simulink model "kumaraGazeboSim2019"  (R2019b)
settings: Solver=FixedStepAuto  StartTime=0.0  StopTime=inf  RelTol=1e-3
model workspace (MAT data in the model file):
  SL_ROS_VariableLengthArrays_MaxSizes.CommonInfo.ArrayTruncateAction = 'EmitWarning'
  SL_ROS_VariableLengthArrays_MaxSizes.MsgTypeMap = containers.Map
  SL_ROS_VariableLengthArrays_MaxSizes.MsgTypeMap.serialization.keys = {'gazebo_msgs/LinkState', 'sensor_msgs/JointState'}
  SL_ROS_VariableLengthArrays_MaxSizes.MsgTypeMap.serialization.values{1}(1).PropertyName = 'LinkName'
  SL_ROS_VariableLengthArrays_MaxSizes.MsgTypeMap.serialization.values{1}(1).DataType = 'uint8'
  SL_ROS_VariableLengthArrays_MaxSizes.MsgTypeMap.serialization.values{1}(1).MaxLength = 18
  SL_ROS_VariableLengthArrays_MaxSizes.MsgTypeMap.serialization.values{1}(2).PropertyName = 'ReferenceFrame'
  SL_ROS_VariableLengthArrays_MaxSizes.MsgTypeMap.serialization.values{1}(2).DataType = 'uint8'
  SL_ROS_VariableLengthArrays_MaxSizes.MsgTypeMap.serialization.values{1}(2).MaxLength = 22
  SL_ROS_VariableLengthArrays_MaxSizes.MsgTypeMap.serialization.values{2}(1).PropertyName = 'Effort'
  SL_ROS_VariableLengthArrays_MaxSizes.MsgTypeMap.serialization.values{2}(1).DataType = 'double'
  SL_ROS_VariableLengthArrays_MaxSizes.MsgTypeMap.serialization.values{2}(1).MaxLength = 13
  SL_ROS_VariableLengthArrays_MaxSizes.MsgTypeMap.serialization.values{2}(2).PropertyName = 'Name'
  SL_ROS_VariableLengthArrays_MaxSizes.MsgTypeMap.serialization.values{2}(2).DataType = 'std_msgs/String'
  SL_ROS_VariableLengthArrays_MaxSizes.MsgTypeMap.serialization.values{2}(2).MaxLength = 13
  SL_ROS_VariableLengthArrays_MaxSizes.MsgTypeMap.serialization.values{2}(3).PropertyName = 'Position'
  SL_ROS_VariableLengthArrays_MaxSizes.MsgTypeMap.serialization.values{2}(3).DataType = 'double'
  SL_ROS_VariableLengthArrays_MaxSizes.MsgTypeMap.serialization.values{2}(3).MaxLength = 13
  SL_ROS_VariableLengthArrays_MaxSizes.MsgTypeMap.serialization.values{2}(4).PropertyName = 'Velocity'
  SL_ROS_VariableLengthArrays_MaxSizes.MsgTypeMap.serialization.values{2}(4).DataType = 'double'
  SL_ROS_VariableLengthArrays_MaxSizes.MsgTypeMap.serialization.values{2}(4).MaxLength = 13
  SL_ROS_VariableLengthArrays_MaxSizes.MsgTypeMap.serialization.uniformity = 0
  SL_ROS_VariableLengthArrays_MaxSizes.MsgTypeMap.serialization.keyType = 'char'
  SL_ROS_VariableLengthArrays_MaxSizes.MsgTypeMap.serialization.valueType = 'any'
libraries: robotlib x21, simulink x3, simulink_extras x2
settings Model: EnablePacing=on  Creator=pokpong.c  LastModifiedBy=pokpong.c
settings OptimizationCC: EnhancedBackFolding=on  PassReuseOutputArgsAs=Individual arguments  ZeroExternalMemoryAtStartup=off  ZeroInternalMemoryAtStartup=off  MaxStackSize=64  OptimizeBlockOrder=speed  DifferentSizesBufferReuse=on  OptimizationCustomize=off  EfficientTunableParamExpr=on
settings DebuggingCC: ParameterTunabilityLossMsg=error
settings HardwareCC: ProdBitPerPointer=32  ProdBitPerSizeT=32  ProdBitPerPtrDiffT=32  ProdLargestAtomicFloat=None  ProdIntDivRoundTo=Undefined  ProdEndianess=Unspecified  ProdWordSize=32  ProdHWDeviceType=Generic->Unspecified (assume 32-bit Generic)
settings SFSimCC: MATLABDynamicMemAlloc=off
settings RTWCC: SystemTargetFile=ert.tlc  HardwareBoard=Robot Operating System (ROS)  TLCOptions="-aInlineSetEventsForThisBaseRateFcn=TLC_FALSE -aSuppressMultiTaskScheduler=TLC_FALSE  -aRateBasedStepFcn=0"  TemplateMakefile=ert_default_tmf  Toolchain=Catkin  TargetLang=C++
settings CodeAppCC: ForceParamTrailComments=on  IgnoreCustomStorageClasses=off  OperatorAnnotations=on  SimulinkDataObjDesc=on  SFDataObjDesc=on  InsertBlockDesc=on

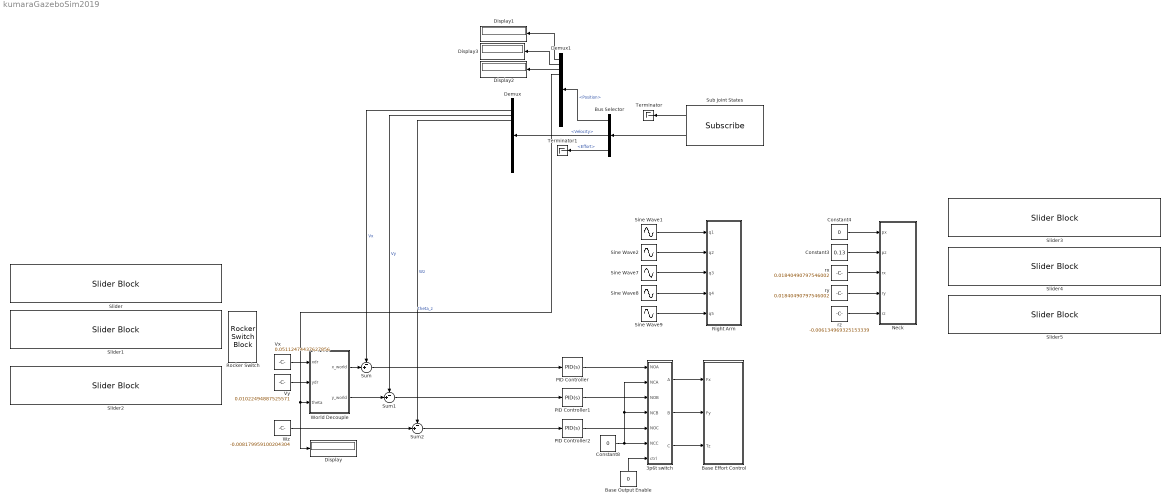
== system kumaraGazeboSim2019 ==
  3p6t switch : Subsystem
  Base Effort Control : Subsystem
  Base Output Enable : Constant  Value=0
  Bus Selector : BusSelector  OutputSignals=Position,Velocity,Effort
  Constant3 : Constant  Value=0.13
  Constant4 : Constant  Value=0
  Constant8 : Constant  Value=0
  Demux : Demux  Outputs=13
  Demux1 : Demux  Outputs=13
  Display{,1..3} (4 alike) : Display
  Neck : Subsystem
  PID Controller : simulink/Continuous/PID Controller  Controller=PID  Form=Parallel  TimeDomain=Continuous-time  SampleTime=-1  IntegratorMethod=Forward Euler  FilterMethod=Forward Euler  ControllerParametersSource=internal  P=40  I=1  D=0  UseFilter=on  N=100  TunerSelectOption=Transfer Function Based (PID Tuner App)  InitialConditionSource=internal  InitialConditionForIntegrator=0  InitialConditionForFilter=0  DifferentiatorICPrevScaledInput=0  ExternalReset=none  TrackingMode=off  Kt=1  LimitOutput=off  UpperSaturationLimit=inf  LowerSaturationLimit=-inf  LinearizeAsGain=on  AntiWindupMode=none  Kb=1  POutMin=[]  POutMax=[]  IOutMin=[]  IOutMax=[]  DOutMin=[]  DOutMax=[]  NOutMin=[]  NOutMax=[]  SumOutMin=[]  SumOutMax=[]  SaturationOutMin=[]  SaturationOutMax=[]  PParamMin=[]  PParamMax=[]  IParamMin=[]  IParamMax=[]  DParamMin=[]  DParamMax=[]  NParamMin=[]  NParamMax=[]  KbParamMin=[]  KbParamMax=[]  KtParamMin=[]  KtParamMax=[]  KbOutMin=[]  KbOutMax=[]  KtOutMin=[]  KtOutMax=[]  IntegratorOutMin=[]  IntegratorOutMax=[]  FilterOutMin=[]  FilterOutMax=[]  SumI1OutMin=[]  SumI1OutMax=[]  SumI2OutMin=[]  SumI2OutMax=[]  SumI3OutMin=[]  SumI3OutMax=[]  SumI4OutMin=[]  SumI4OutMax=[]  SumDOutMin=[]  SumDOutMax=[]  DifferentiatorOutMin=[]  DifferentiatorOutMax=[]  FilterDiffOutCoefMin=[]  FilterDiffOutCoefMax=[]  ReciprocalOutMin=[]  ReciprocalOutMax=[]  SumDenOutMin=[]  SumDenOutMax=[]  SumNumOutMin=[]  SumNumOutMax=[]  DivideOutMin=[]  DivideOutMax=[]  IntegratorContinuousStateAttributes=''  IntegratorStateMustResolveToSignalObject=off  IntegratorRTWStateStorageClass=Auto  FilterContinuousStateAttributes=''  FilterStateMustResolveToSignalObject=off  FilterRTWStateStorageClass=Auto  ParallelPVariant=InternalParameters  IdealPVariant=Disabled  IVariant=InternalParameters  DVariant=InternalParameters  IntegratorVariant=Continuous  SatVariant=Disabled  AWVariant=Passthrough  PCopyVariant=Disabled  TRVariant=Disabled  FdbkBlocksVariant=Forward  IdealPFdbkVariant=Disabled  SatFdbkVariant=Disabled  DerivativeFilterVariant=ContFilter  NVariant=InternalParameters  NCopyVariant=Disabled  FilterICVariant=InternalICsFilter  IntegratorICVariant=InternalICs  ExternalResetVariant=Disabled  TRSumVariant=Passthrough  SumFdbkVariant=Disabled  SumVariant=Sum_PID
  PID Controller1 : simulink/Continuous/PID Controller  Controller=PID  Form=Parallel  TimeDomain=Continuous-time  SampleTime=-1  IntegratorMethod=Forward Euler  FilterMethod=Forward Euler  ControllerParametersSource=internal  P=40  I=1  D=0  UseFilter=on  N=100  TunerSelectOption=Transfer Function Based (PID Tuner App)  InitialConditionSource=internal  InitialConditionForIntegrator=0  InitialConditionForFilter=0  DifferentiatorICPrevScaledInput=0  ExternalReset=none  TrackingMode=off  Kt=1  LimitOutput=off  UpperSaturationLimit=inf  LowerSaturationLimit=-inf  LinearizeAsGain=on  AntiWindupMode=none  Kb=1  POutMin=[]  POutMax=[]  IOutMin=[]  IOutMax=[]  DOutMin=[]  DOutMax=[]  NOutMin=[]  NOutMax=[]  SumOutMin=[]  SumOutMax=[]  SaturationOutMin=[]  SaturationOutMax=[]  PParamMin=[]  PParamMax=[]  IParamMin=[]  IParamMax=[]  DParamMin=[]  DParamMax=[]  NParamMin=[]  NParamMax=[]  KbParamMin=[]  KbParamMax=[]  KtParamMin=[]  KtParamMax=[]  KbOutMin=[]  KbOutMax=[]  KtOutMin=[]  KtOutMax=[]  IntegratorOutMin=[]  IntegratorOutMax=[]  FilterOutMin=[]  FilterOutMax=[]  SumI1OutMin=[]  SumI1OutMax=[]  SumI2OutMin=[]  SumI2OutMax=[]  SumI3OutMin=[]  SumI3OutMax=[]  SumI4OutMin=[]  SumI4OutMax=[]  SumDOutMin=[]  SumDOutMax=[]  DifferentiatorOutMin=[]  DifferentiatorOutMax=[]  FilterDiffOutCoefMin=[]  FilterDiffOutCoefMax=[]  ReciprocalOutMin=[]  ReciprocalOutMax=[]  SumDenOutMin=[]  SumDenOutMax=[]  SumNumOutMin=[]  SumNumOutMax=[]  DivideOutMin=[]  DivideOutMax=[]  IntegratorContinuousStateAttributes=''  IntegratorStateMustResolveToSignalObject=off  IntegratorRTWStateStorageClass=Auto  FilterContinuousStateAttributes=''  FilterStateMustResolveToSignalObject=off  FilterRTWStateStorageClass=Auto  ParallelPVariant=InternalParameters  IdealPVariant=Disabled  IVariant=InternalParameters  DVariant=InternalParameters  IntegratorVariant=Continuous  SatVariant=Disabled  AWVariant=Passthrough  PCopyVariant=Disabled  TRVariant=Disabled  FdbkBlocksVariant=Forward  IdealPFdbkVariant=Disabled  SatFdbkVariant=Disabled  DerivativeFilterVariant=ContFilter  NVariant=InternalParameters  NCopyVariant=Disabled  FilterICVariant=InternalICsFilter  IntegratorICVariant=InternalICs  ExternalResetVariant=Disabled  TRSumVariant=Passthrough  SumFdbkVariant=Disabled  SumVariant=Sum_PID
  PID Controller2 : simulink/Continuous/PID Controller  Controller=PID  Form=Parallel  TimeDomain=Continuous-time  SampleTime=-1  IntegratorMethod=Forward Euler  FilterMethod=Forward Euler  ControllerParametersSource=internal  P=40  I=1  D=0  UseFilter=on  N=100  TunerSelectOption=Transfer Function Based (PID Tuner App)  InitialConditionSource=internal  InitialConditionForIntegrator=0  InitialConditionForFilter=0  DifferentiatorICPrevScaledInput=0  ExternalReset=none  TrackingMode=off  Kt=1  LimitOutput=off  UpperSaturationLimit=inf  LowerSaturationLimit=-inf  LinearizeAsGain=on  AntiWindupMode=none  Kb=1  POutMin=[]  POutMax=[]  IOutMin=[]  IOutMax=[]  DOutMin=[]  DOutMax=[]  NOutMin=[]  NOutMax=[]  SumOutMin=[]  SumOutMax=[]  SaturationOutMin=[]  SaturationOutMax=[]  PParamMin=[]  PParamMax=[]  IParamMin=[]  IParamMax=[]  DParamMin=[]  DParamMax=[]  NParamMin=[]  NParamMax=[]  KbParamMin=[]  KbParamMax=[]  KtParamMin=[]  KtParamMax=[]  KbOutMin=[]  KbOutMax=[]  KtOutMin=[]  KtOutMax=[]  IntegratorOutMin=[]  IntegratorOutMax=[]  FilterOutMin=[]  FilterOutMax=[]  SumI1OutMin=[]  SumI1OutMax=[]  SumI2OutMin=[]  SumI2OutMax=[]  SumI3OutMin=[]  SumI3OutMax=[]  SumI4OutMin=[]  SumI4OutMax=[]  SumDOutMin=[]  SumDOutMax=[]  DifferentiatorOutMin=[]  DifferentiatorOutMax=[]  FilterDiffOutCoefMin=[]  FilterDiffOutCoefMax=[]  ReciprocalOutMin=[]  ReciprocalOutMax=[]  SumDenOutMin=[]  SumDenOutMax=[]  SumNumOutMin=[]  SumNumOutMax=[]  DivideOutMin=[]  DivideOutMax=[]  IntegratorContinuousStateAttributes=''  IntegratorStateMustResolveToSignalObject=off  IntegratorRTWStateStorageClass=Auto  FilterContinuousStateAttributes=''  FilterStateMustResolveToSignalObject=off  FilterRTWStateStorageClass=Auto  ParallelPVariant=InternalParameters  IdealPVariant=Disabled  IVariant=InternalParameters  DVariant=InternalParameters  IntegratorVariant=Continuous  SatVariant=Disabled  AWVariant=Passthrough  PCopyVariant=Disabled  TRVariant=Disabled  FdbkBlocksVariant=Forward  IdealPFdbkVariant=Disabled  SatFdbkVariant=Disabled  DerivativeFilterVariant=ContFilter  NVariant=InternalParameters  NCopyVariant=Disabled  FilterICVariant=InternalICsFilter  IntegratorICVariant=InternalICs  ExternalResetVariant=Disabled  TRSumVariant=Passthrough  SumFdbkVariant=Disabled  SumVariant=Sum_PID
  Right Arm : Subsystem
  Rocker Switch : RockerSwitchBlock
      settings: Values={{'Off', 'On'}, [0 1]}
  Sine Wave{1..2,7..9} (5 alike) : Sin  Amplitude=3  Frequency=3  SampleTime=0
  Slider : SliderBlock  ScaleMin=-5  ScaleMax=5
  Slider1 : SliderBlock  ScaleMin=-5  ScaleMax=5
  Slider2 : SliderBlock  ScaleMin=-4  ScaleMax=4
  Slider3 : SliderBlock  ScaleMin=-3  ScaleMax=3
  Slider4 : SliderBlock  ScaleMin=-3  ScaleMax=3
  Slider5 : SliderBlock  ScaleMin=-3  ScaleMax=3
  Sub Joint States : robotlib/Subscribe  topicSource=Select from ROS network  topic=/kumara/joint_states  messageType=sensor_msgs/JointState  sampleTime=0.01  messageQueueLength=1
  Sum : Sum  Inputs=-+|
  Sum1 : Sum  Inputs=-+|
  Sum2 : Sum  Inputs=-+|
  Terminator : Terminator
  Terminator1 : Terminator
  Vx : Constant  Value=0.05112474437627856
  Vy : Constant  Value=0.01022494887525571
  World Decouple : Subsystem
  Wz : Constant  Value=-0.008179959100204304
  rx : Constant  Value=0.01840490797546002
  ry : Constant  Value=0.01840490797546002
  rz : Constant  Value=-0.006134969325153339
  wires:
  Vx/1 -> World Decouple/1("xdr ")
  Bus Selector/1 -> Demux1/1  "<Position>"
  Demux1/4 -> Display/1, World Decouple/3("theta ")  "theta_z"
  World Decouple/1(x_world) -> Sum/2
  World Decouple/2(y_world) -> Sum1/2
  PID Controller/1 -> 3p6t switch/1(NOA)
  Demux/4 -> Sum2/1  "Wz"
  Sum/1 -> PID Controller/1
  Base Output Enable/1 -> 3p6t switch/7(ctrl)
  Constant8/1 -> 3p6t switch/6(NCC), 3p6t switch/4(NCB), 3p6t switch/2(NCA)
  3p6t switch/1(A) -> Base Effort Control/1(Fx)
  Sub Joint States/2 -> Bus Selector/1
  Bus Selector/2 -> Demux/1  "<Velocity>"
  Vy/1 -> World Decouple/2(ydr)
  3p6t switch/3(C) -> Base Effort Control/3(Tz)
  Sum2/1 -> PID Controller2/1
  PID Controller1/1 -> 3p6t switch/3(NOB)
  Demux/3 -> Sum1/1  "Vy"
  Demux/2 -> Sum/1  "Vx"
  PID Controller2/1 -> 3p6t switch/5(NOC)
  Wz/1 -> Sum2/2
  Sum1/1 -> PID Controller1/1
  Sub Joint States/1 -> Terminator/1
  3p6t switch/2(B) -> Base Effort Control/2(Fy)
  Bus Selector/3 -> Terminator1/1  "<Effort>"
  Constant3/1 -> Neck/2(pz)
  Demux1/1 -> Display1/1
  Demux1/3 -> Display2/1
  Demux1/2 -> Display3/1
  Sine Wave1/1 -> Right Arm/1(q1)
  Sine Wave2/1 -> Right Arm/2(q2)
  Sine Wave7/1 -> Right Arm/3(q3)
  Sine Wave8/1 -> Right Arm/4(q4)
  Sine Wave9/1 -> Right Arm/5(q5)
  Constant4/1 -> Neck/1(px)
  rx/1 -> Neck/3(rx)
  ry/1 -> Neck/4(ry)
  rz/1 -> Neck/5(rz)

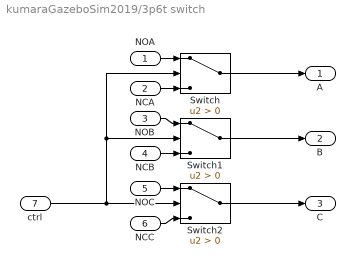
== system kumaraGazeboSim2019/3p6t switch ==
  NOA : Inport
  NCA : Inport  Port=2
  NOB : Inport  Port=3
  NCB : Inport  Port=4
  NOC : Inport  Port=5
  NCC : Inport  Port=6
  ctrl : Inport  Port=7
  Switch : Switch  Criteria=u2 > Threshold
  Switch1 : Switch  Criteria=u2 > Threshold
  Switch2 : Switch  Criteria=u2 > Threshold
  A : Outport
  B : Outport  Port=2
  C : Outport  Port=3
  wires:
  Switch1/1 -> B/1
  NCB/1 -> Switch1/3
  Switch/1 -> A/1
  NCC/1 -> Switch2/3
  Switch2/1 -> C/1
  ctrl/1 -> Switch2/2, Switch/2, Switch1/2
  NOA/1 -> Switch/1
  NOB/1 -> Switch1/1
  NCA/1 -> Switch/3
  NOC/1 -> Switch2/1

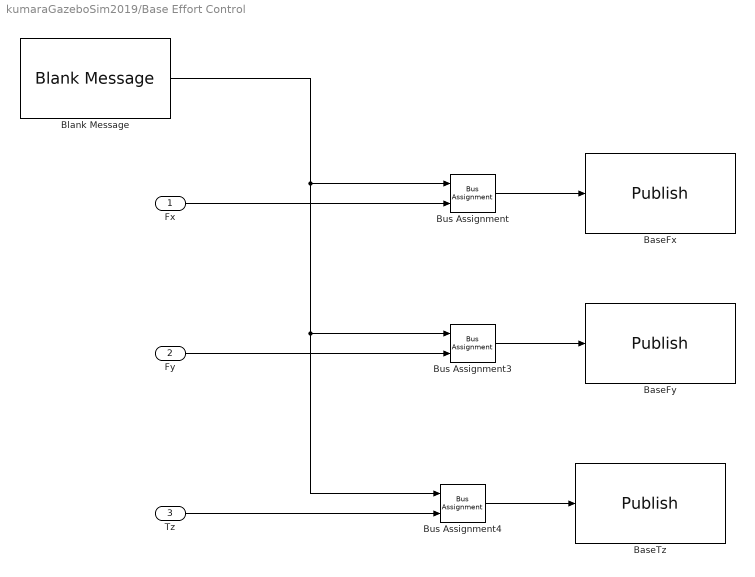
== system kumaraGazeboSim2019/Base Effort Control ==
  Fx : Inport
  Fy : Inport  Port=2
  Tz : Inport  Port=3
  BaseFx : robotlib/Publish  topicSource=Select from ROS network  topic=/kumara/base_x_force_controller/command  messageType=std_msgs/Float64  messageQueueLength=1
  BaseFy : robotlib/Publish  topicSource=Select from ROS network  topic=/kumara/base_y_force_controller/command  messageType=std_msgs/Float64  messageQueueLength=1
  BaseTz : robotlib/Publish  topicSource=Select from ROS network  topic=/kumara/base_z_torque_controller/command  messageType=std_msgs/Float64  messageQueueLength=1
  Blank Message : robotlib/Blank Message  messageClass=Message  entityType=std_msgs/Float64  messageType=std_msgs/Float64  SampleTime=inf
  Bus Assignment : BusAssignment  AssignedSignals=Data
  Bus Assignment3 : BusAssignment  AssignedSignals=Data
  Bus Assignment4 : BusAssignment  AssignedSignals=Data
  wires:
  Bus Assignment/1 -> BaseFx/1
  Bus Assignment3/1 -> BaseFy/1
  Bus Assignment4/1 -> BaseTz/1
  Blank Message/1 -> Bus Assignment/1, Bus Assignment3/1, Bus Assignment4/1
  Tz/1 -> Bus Assignment4/2
  Fx/1 -> Bus Assignment/2
  Fy/1 -> Bus Assignment3/2

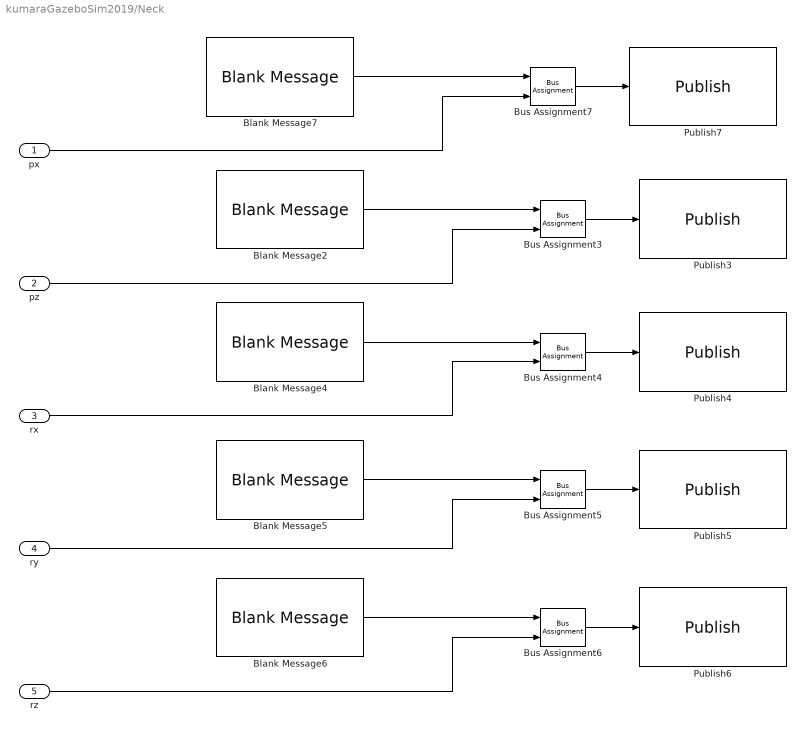
== system kumaraGazeboSim2019/Neck ==
  px : Inport
  pz : Inport  Port=2
  rx : Inport  Port=3
  ry : Inport  Port=4
  rz : Inport  Port=5
  Blank Message{2,4..7} (5 alike) : robotlib/Blank Message  messageClass=Message  entityType=std_msgs/Float64  messageType=std_msgs/Float64  SampleTime=inf
  Bus Assignment{3..7} (5 alike) : BusAssignment  AssignedSignals=Data
  Publish3 : robotlib/Publish  topicSource=Select from ROS network  topic=/kumara/neck_z_position_controller/command  messageType=std_msgs/Float64  messageQueueLength=1
  Publish4 : robotlib/Publish  topicSource=Select from ROS network  topic=/kumara/neck_rx_position_controller/command  messageType=std_msgs/Float64  messageQueueLength=1
  Publish5 : robotlib/Publish  topicSource=Select from ROS network  topic=/kumara/neck_ry_position_controller/command  messageType=std_msgs/Float64  messageQueueLength=1
  Publish6 : robotlib/Publish  topicSource=Select from ROS network  topic=/kumara/neck_rz_position_controller/command  messageType=std_msgs/Float64  messageQueueLength=1
  Publish7 : robotlib/Publish  topicSource=Select from ROS network  topic=/kumara/neck_x_position_controller/command  messageType=std_msgs/Float64  messageQueueLength=1
  wires:
  Blank Message6/1 -> Bus Assignment6/1
  Blank Message5/1 -> Bus Assignment5/1
  Blank Message7/1 -> Bus Assignment7/1
  Bus Assignment6/1 -> Publish6/1
  Bus Assignment7/1 -> Publish7/1
  Bus Assignment3/1 -> Publish3/1
  Blank Message2/1 -> Bus Assignment3/1
  Bus Assignment4/1 -> Publish4/1
  Bus Assignment5/1 -> Publish5/1
  Blank Message4/1 -> Bus Assignment4/1
  px/1 -> Bus Assignment7/2
  pz/1 -> Bus Assignment3/2
  ry/1 -> Bus Assignment5/2
  rx/1 -> Bus Assignment4/2
  rz/1 -> Bus Assignment6/2

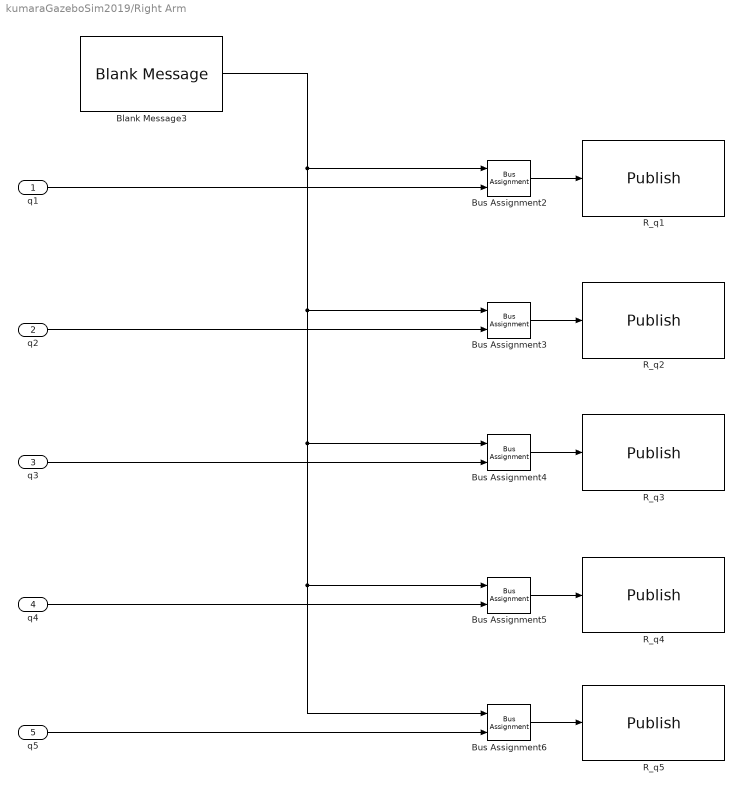
== system kumaraGazeboSim2019/Right Arm ==
  q1 : Inport
  q2 : Inport  Port=2
  q3 : Inport  Port=3
  q4 : Inport  Port=4
  q5 : Inport  Port=5
  Blank Message3 : robotlib/Blank Message  messageClass=Message  entityType=std_msgs/Float64  messageType=std_msgs/Float64  SampleTime=inf
  Bus Assignment{2..6} (5 alike) : BusAssignment  AssignedSignals=Data
  R_q1 : robotlib/Publish  topicSource=Select from ROS network  topic=/kumara/r_arm_q1_torque_controller/command  messageType=std_msgs/Float64  messageQueueLength=1
  R_q2 : robotlib/Publish  topicSource=Select from ROS network  topic=/kumara/r_arm_q2_torque_controller/command  messageType=std_msgs/Float64  messageQueueLength=1
  R_q3 : robotlib/Publish  topicSource=Select from ROS network  topic=/kumara/r_arm_q3_torque_controller/command  messageType=std_msgs/Float64  messageQueueLength=1
  R_q4 : robotlib/Publish  topicSource=Select from ROS network  topic=/kumara/r_arm_q4_torque_controller/command  messageType=std_msgs/Float64  messageQueueLength=1
  R_q5 : robotlib/Publish  topicSource=Select from ROS network  topic=/kumara/r_arm_q5_torque_controller/command  messageType=std_msgs/Float64  messageQueueLength=1
  wires:
  q4/1 -> Bus Assignment5/2
  Blank Message3/1 -> Bus Assignment2/1, Bus Assignment3/1, Bus Assignment5/1, Bus Assignment6/1, Bus Assignment4/1
  Bus Assignment2/1 -> R_q1/1
  Bus Assignment4/1 -> R_q3/1
  q2/1 -> Bus Assignment3/2
  Bus Assignment6/1 -> R_q5/1
  Bus Assignment5/1 -> R_q4/1
  Bus Assignment3/1 -> R_q2/1
  q1/1 -> Bus Assignment2/2
  q5/1 -> Bus Assignment6/2
  q3/1 -> Bus Assignment4/2

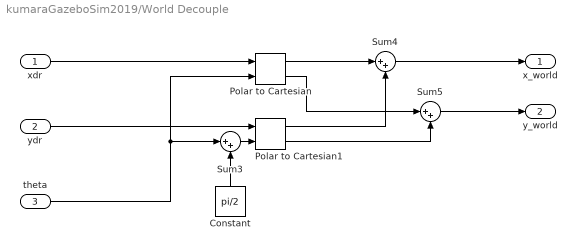
== system kumaraGazeboSim2019/World Decouple ==
  "xdr " : Inport
  ydr : Inport  Port=2
  "theta " : Inport  Port=3
  Constant : Constant  Value=pi/2
  Polar to Cartesian : simulink_extras/Transformations/Polar to Cartesian
      settings: SourceProductBaseCode=SL
  Polar to Cartesian1 : simulink_extras/Transformations/Polar to Cartesian
      settings: SourceProductBaseCode=SL
  Sum3 : Sum  Inputs=|++
  Sum4 : Sum  Inputs=|++
  Sum5 : Sum  Inputs=|++
  x_world : Outport
  y_world : Outport  Port=2
  wires:
  "theta "/1 -> Sum3/1, Polar to Cartesian/2
  Constant/1 -> Sum3/2
  ydr/1 -> Polar to Cartesian1/1
  Sum3/1 -> Polar to Cartesian1/2
  Polar to Cartesian1/1 -> Sum4/2
  Sum4/1 -> x_world/1
  Polar to Cartesian/1 -> Sum4/1
  Polar to Cartesian/2 -> Sum5/1
  Polar to Cartesian1/2 -> Sum5/2
  Sum5/1 -> y_world/1
  "xdr "/1 -> Polar to Cartesian/1
